simulink model "autosar_swc"  (R2021a)
settings: Solver=FixedStepAuto  StartTime=0.0  StopTime=10.0  RelTol=1e-3  EnableMultiTasking=on
undefined symbols (not defined in the file): DiscIntNeverNeededParam
settings Model: Creator=yangpeihao  LastModifiedBy=ASUS
settings OptimizationCC: DefaultParameterBehavior=Inlined  UseDivisionForNetSlopeComputation=on  GainParamInheritBuiltInType=on  UseFloatMulNetSlope=on  InlineInvariantSignals=on  PassReuseOutputArgsAs=Individual arguments  ZeroExternalMemoryAtStartup=off  ZeroInternalMemoryAtStartup=off  NoFixptDivByZeroProtection=on  EfficientFloat2IntCast=on  LifeSpan=1  OptimizeBlockOrder=speed  DifferentSizesBufferReuse=on  EfficientTunableParamExpr=on
settings DebuggingCC: ParameterTunabilityLossMsg=error
settings HardwareCC: ProdLongLongMode=on
settings SFSimCC: MATLABDynamicMemAlloc=off
settings RTWCC: Description=AUTOSAR  SystemTargetFile=autosar.tlc  GenCodeOnly=on  TemplateMakefile=ert_default_tmf
settings CodeAppCC: ForceParamTrailComments=on  IgnoreCustomStorageClasses=off  OperatorAnnotations=on  SimulinkDataObjDesc=on  SFDataObjDesc=on  CustomSymbolStrGlobalVar=rt$N$M  CustomSymbolStrType=$N$M  CustomSymbolStrFcn=$N$M$F  CustomSymbolStrMacro=$N$M  InsertBlockDesc=on
settings STFCustomTargetCC: TargetLangStandard=C99 (ISO)  MultiwordLength=256  ParMdlRefBuildCompliant=on  CompOptLevelCompliant=on  IncludeMdlTerminateFcn=off  CombineOutputUpdateFcns=on  CombineSignalStateStructs=on  SuppressErrorStatus=on  ERTCustomFileBanners=on  SupportAbsoluteTime=off  SupportNonFinite=off  SupportComplex=off  SupportContinuousTime=off  SupportNonInlinedSFcns=off  RemoveResetFunc=on  MATLABClassNameForMDSCustomization=Simulink.SoftwareTarget.ERTCustomization  AutosarCompliant=on  GRTInterface=off  LookupTableObjectStructAxisOrder=2,1,3,4,...  LUTObjectStructOrderEvenSpacing=Size,Table,Breakpoints  SystemTargetFile=autosar.tlc
settings ERTTargetCC: TargetLangStandard=C99 (ISO)  ConcurrentExecutionCompliant=off  IncludeMdlTerminateFcn=off  CombineSignalStateStructs=on  SuppressErrorStatus=on  SupportAbsoluteTime=off  SupportNonFinite=off  SupportComplex=off  ModelStepFunctionPrototypeControlCompliant=off  CPPClassGenCompliant=off  AutosarCompliant=on  LookupTableObjectStructAxisOrder=2,1,3,4,...  LUTObjectStructOrderEvenSpacing=Size,Table,Breakpoints  InlinedParameterPlacement=NonHierarchical  ERTCustomFileTemplate=example_file_process.tlc  ERTFilePackagingFormat=CompactWithDataFile

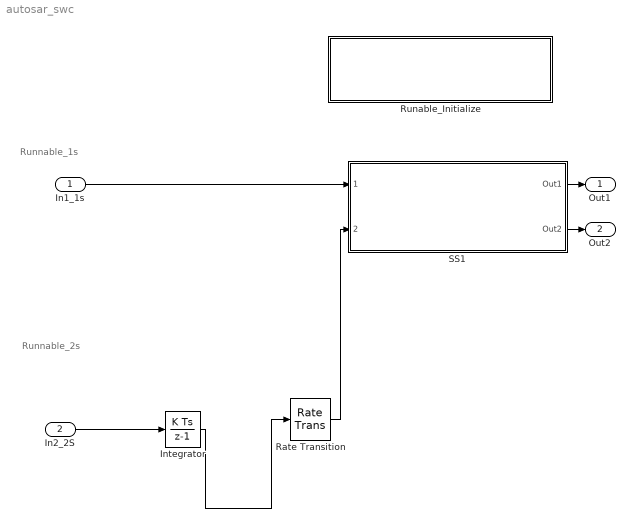
== system autosar_swc ==
  note: Runnable_2s
  note: Runnable_1s
  In1_1s : Inport  OutDataTypeStr=double  PortDimensions=1  SampleTime=1
  In2_2S : Inport  Port=2  SampleTime=2
  Integrator : DiscreteIntegrator  SampleTime=-1  SaturateOnIntegerOverflow=on  ICPrevOutput=DiscIntNeverNeededParam  ICPrevScaledInput=DiscIntNeverNeededParam
  Rate Transition : RateTransition  Deterministic=off
  Runable_Initialize : Subsystem  TreatAsAtomicUnit=on
  SS1 : Subsystem
  Out1 : Outport
  Out2 : Outport  Port=2
  wires:
  In2_2S/1 -> Integrator/1
  Integrator/1 -> Rate Transition/1
  In1_1s/1 -> SS1/1(1)
  SS1/1(Out1) -> Out1/1
  SS1/2(Out2) -> Out2/1
  Rate Transition/1 -> SS1/2(2)

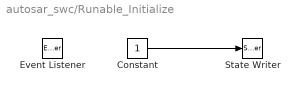
== system autosar_swc/Runable_Initialize ==
  Constant : Constant
  Event Listener : EventListener  DisableCoverage=on  EventName=reset
  State Writer : StateWriter  StateOwnerBlock=../../Integrator
  wires:
  Constant/1 -> State Writer/1

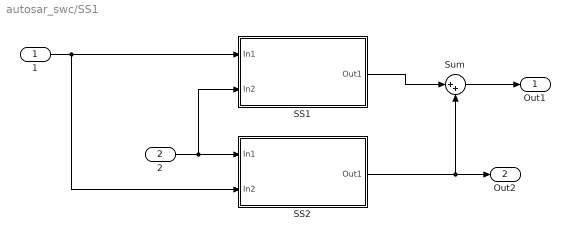
== system autosar_swc/SS1 ==
  1 : Inport
  2 : Inport  Port=2
  SS1 : Subsystem
  SS2 : Subsystem
  Sum : Sum  Inputs=|++
  Out1 : Outport
  Out2 : Outport  Port=2
  wires:
  1/1 -> SS2/2(In2), SS1/1(In1)
  2/1 -> SS1/2(In2), SS2/1(In1)
  SS2/1(Out1) -> Sum/2, Out2/1
  Sum/1 -> Out1/1
  SS1/1(Out1) -> Sum/1

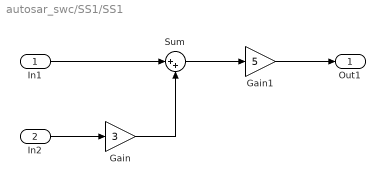
== system autosar_swc/SS1/SS1 ==
  In1 : Inport
  In2 : Inport  Port=2
  Gain : Gain  Gain=3  OutDataTypeStr=Inherit: Same as input  ParamDataTypeStr=Inherit: Same as input
  Gain1 : Gain  Gain=5  OutDataTypeStr=Inherit: Same as input  ParamDataTypeStr=Inherit: Same as input
  Sum : Sum  Inputs=|++  OutDataTypeStr=Inherit: Same as first input
  Out1 : Outport
  wires:
  In2/1 -> Gain/1
  In1/1 -> Sum/1
  Gain/1 -> Sum/2
  Sum/1 -> Gain1/1
  Gain1/1 -> Out1/1

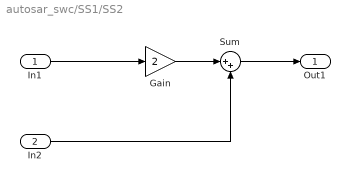
== system autosar_swc/SS1/SS2 ==
  In1 : Inport
  In2 : Inport  Port=2
  Gain : Gain  Gain=2  OutDataTypeStr=Inherit: Same as input  ParamDataTypeStr=Inherit: Same as input
  Sum : Sum  Inputs=|++
  Out1 : Outport
  wires:
  In1/1 -> Gain/1
  Gain/1 -> Sum/1
  Sum/1 -> Out1/1
  In2/1 -> Sum/2
